simulink model "final_1EHA_comfiltro_V9"  (R2016a)
settings: Solver=FixedStepAuto  StartTime=72.65  StopTime=73.9  FixedStep=Ts  MaxStep=1e-7  RelTol=1e-4  AbsTol=1e-4
PreLoadFcn:
  | % -- Recommended Settings --
  | %
  | %  Simulink:
  | %      Solver: Ode23t
  | %      Relative tolerance = 1e-3
  | %       Max step size = 0.2
  | %
  | %  Powergui:
  |          Ts = 1e-07; % (discrete electrical model)
  | %
  | %  Control systems:
  |          Ts_control = 10*Ts; % (discrete control system)
  | %
  | % ----------------------------------
undefined symbols (not defined in the file or in its folder): C, L, R1, R2, sigbuilder_block
libraries: powerlib x92, dsparch4 x12, simulink x6, sps_avr x1, powerlib_meascontrol x1
(part 2 of 2)

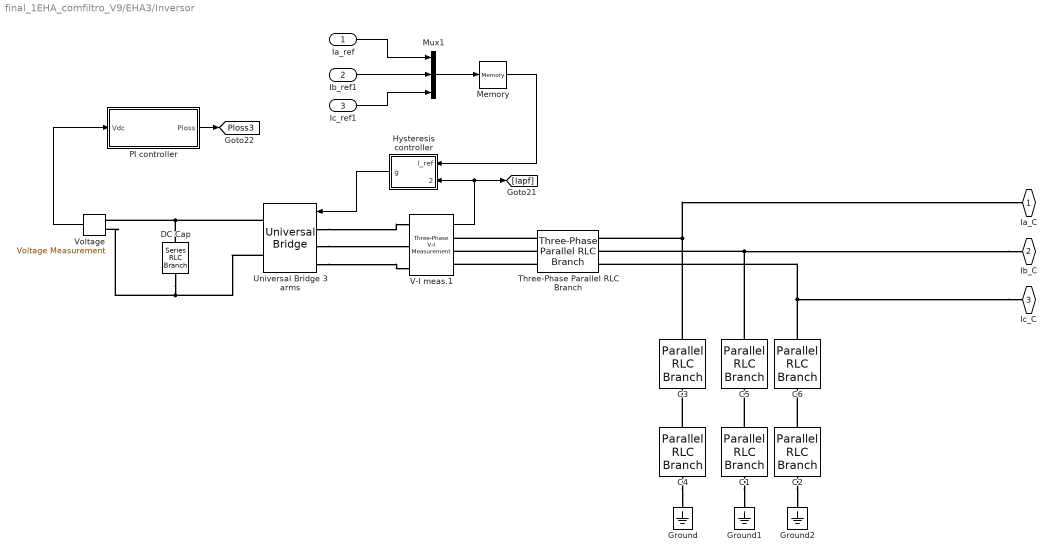
== system final_1EHA_comfiltro_V9/EHA3/Inversor ==
  Ia_ref : Inport
  Ib_ref1 : Inport  Port=2
  Ic_ref1 : Inport  Port=3
  C1 : powerlib/Elements/Parallel RLC Branch  LConnTagsString=a  RConnTagsString=__new0  BranchType=RC  Resistance=R2  Inductance=1e-3  SetiL0=off  InitialCurrent=0  Capacitance=C  Setx0=off  InitialVoltage=0  Measurements=None
  C2 : powerlib/Elements/Parallel RLC Branch  LConnTagsString=a  RConnTagsString=__new0  BranchType=RC  Resistance=R2  Inductance=1e-3  SetiL0=off  InitialCurrent=0  Capacitance=C  Setx0=off  InitialVoltage=0  Measurements=None
  C3 : powerlib/Elements/Parallel RLC Branch  LConnTagsString=a  RConnTagsString=__new0  BranchType=R  Resistance=R1  Inductance=1e-3  SetiL0=off  InitialCurrent=0  Capacitance=C  Setx0=off  InitialVoltage=0  Measurements=None
  C4 : powerlib/Elements/Parallel RLC Branch  LConnTagsString=a  RConnTagsString=__new0  BranchType=RC  Resistance=R2  Inductance=1e-3  SetiL0=off  InitialCurrent=0  Capacitance=C  Setx0=off  InitialVoltage=0  Measurements=None
  C5 : powerlib/Elements/Parallel RLC Branch  LConnTagsString=a  RConnTagsString=__new0  BranchType=R  Resistance=R1  Inductance=1e-3  SetiL0=off  InitialCurrent=0  Capacitance=C  Setx0=off  InitialVoltage=0  Measurements=None
  C6 : powerlib/Elements/Parallel RLC Branch  LConnTagsString=a  RConnTagsString=__new0  BranchType=R  Resistance=R1  Inductance=1e-3  SetiL0=off  InitialCurrent=0  Capacitance=C  Setx0=off  InitialVoltage=0  Measurements=None
  DC Cap : powerlib/Elements/Series RLC Branch  LConnTagsString=__new0  RConnTagsString=__new0  BranchType=C  Resistance=1  Inductance=1e-3  SetiL0=off  InitialCurrent=0  Capacitance=200e-6  Setx0=off  InitialVoltage=350  Measurements=None
  Ground : powerlib/Elements/Ground  LConnTagsString=a
  Ground1 : powerlib/Elements/Ground  LConnTagsString=a
  Ground2 : powerlib/Elements/Ground  LConnTagsString=a
  Hysteresis controller : Subsystem
  Memory : Memory
  Mux1 : Mux  Inputs=3
  PI controller : Subsystem
  Three-Phase Parallel RLC Branch : powerlib/Elements/Three-Phase Parallel RLC Branch  LConnTagsString=A|B|C  RConnTagsString=A|B|C  BranchType=L  Resistance=1  Inductance=L  Capacitance=1e-6  Measurements=None
  Universal Bridge 3 arms : powerlib/Power Electronics/Universal Bridge  Arms=3  SnubberResistance=1e8  SnubberCapacitance=inf  Device=Ideal Switches  Ron=1e-5  Lon=0  ForwardVoltages="[  1  1  ]"  ForwardVoltage=.8  GTOparameters=[ 10e-6 , 20e-6 ]  IGBTparameters=[ 1e-6 , 2e-6 ]  Measurements=None  Measurements_2=None  converterType=Rectifier
  V-I meas.1 : powerlib/Measurements/Three-Phase V-I Measurement  VoltageMeasurement=no  SetLabelV=off  LabelV=Vnm_EHA1  Vpu=off  VpuLL=off  CurrentMeasurement=yes  SetLabelI=off  LabelI=Iabc  Ipu=off  Pbase=100e6  Vbase=500e3  OutputType=Complex  PhasorSimulation=off  PSBequivalent=0
  Voltage : powerlib/Measurements/Voltage Measurement  PhasorSimulation=off  OutputType=Complex  PSBequivalent=0
  Ia_C : PMIOPort  Port=1  Side=Right
  Ib_C : PMIOPort  Port=2  Side=Right
  Ic_C : PMIOPort  Port=3  Side=Right
  tag scope: Ploss3=global
  wires:
  Voltage/1 -> PI controller/1(Vdc)
  PI controller/1(Ploss) -> [Ploss3]
  V-I meas.1/1 -> Hysteresis controller/2(I_meas), [Iapf]
  Mux1/1 -> Memory/1
  Hysteresis controller/1(g) -> Universal Bridge 3 arms/1
  Ia_ref/1 -> Mux1/1
  Ib_ref1/1 -> Mux1/2
  Ic_ref1/1 -> Mux1/3
  Memory/1 -> Hysteresis controller/1(I_ref)
  connections:
  Voltage/LConn1 -- Universal Bridge 3 arms/RConn1 -- DC Cap/LConn1
  Voltage/LConn2 -- Universal Bridge 3 arms/RConn2 -- DC Cap/RConn1
  Three-Phase Parallel RLC Branch/LConn2 -- V-I meas.1/RConn2
  Universal Bridge 3 arms/LConn1 -- V-I meas.1/LConn1
  Three-Phase Parallel RLC Branch/LConn1 -- V-I meas.1/RConn1
  Universal Bridge 3 arms/LConn2 -- V-I meas.1/LConn2
  Three-Phase Parallel RLC Branch/LConn3 -- V-I meas.1/RConn3
  Universal Bridge 3 arms/LConn3 -- V-I meas.1/LConn3
  Three-Phase Parallel RLC Branch/RConn1 -- C3/LConn1 -- Ia_C/RConn1
  Ib_C/RConn1 -- C5/LConn1 -- Three-Phase Parallel RLC Branch/RConn2
  Ic_C/RConn1 -- C6/LConn1 -- Three-Phase Parallel RLC Branch/RConn3
  C4/RConn1 -- Ground/LConn1
  C4/LConn1 -- C3/RConn1
  C2/LConn1 -- C6/RConn1
  C2/RConn1 -- Ground2/LConn1
  C1/LConn1 -- C5/RConn1
  C1/RConn1 -- Ground1/LConn1

== system final_1EHA_comfiltro_V9/EHA3/Signal Builder ==
  Demux : Demux  Tag=STV Demux  Outputs=1
  FromWs : FromWorkspace  Tag=STV FromWs  VariableName=tuvar  SampleTime=0
      SigBuilderData=|
      | common.afterFinalStr = 'Extrapolate'
      | common.sampleTime = 0
      | dataSet.timeRange = [72.75 73.9]
      | dataSet.name = 'Imported_Group 1'
      | sbobj.Name = 'Signal Builder'
      | sbobj.Groups.Name = 'Imported_Group 1'
      | sbobj.Groups.Signals.Name = 'var'
      | sbobj.Groups.Signals.XData = [72.75 72.751 72.752 72.753 72.754 72.755 72.756 72.757 72.758 72.759 72.76 72.761 ... (1151 elements, 1x1151)]
      | sbobj.Groups.Signals.YData = [0 0 0 0 0 0 0 0 0 0 0 0 ... (1151 elements, 1x1151)]
      | sbobj.Groups.TimeRange = [72.75 73.9]
  var : Outport
  wires:
  Demux/1 -> var/1
  FromWs/1 -> Demux/1

== system final_1EHA_comfiltro_V9/Primary Distribution (measurements & main contactor)/Contactor ==
  com : Inport
  Ideal Switch : powerlib/Power Electronics/Ideal Switch  Ron=0.001  Lon=0  IC=0  Rs=1e3  Cs=inf  Measurements=off
  Ideal Switch1 : powerlib/Power Electronics/Ideal Switch  Ron=0.001  Lon=0  IC=0  Rs=1e3  Cs=inf  Measurements=off
  Ideal Switch2 : powerlib/Power Electronics/Ideal Switch  Ron=0.001  Lon=0  IC=0  Rs=1e3  Cs=inf  Measurements=off
  A : PMIOPort  Port=1  Side=Left
  a : PMIOPort  Port=2  Side=Right
  B : PMIOPort  Port=3  Side=Left
  b : PMIOPort  Port=4  Side=Right
  C : PMIOPort  Port=5  Side=Left
  c : PMIOPort  Port=6  Side=Right
  wires:
  com/1 -> Ideal Switch1/1, Ideal Switch2/1, Ideal Switch/1
  connections:
  c/RConn1 -- Ideal Switch2/RConn1
  C/RConn1 -- Ideal Switch2/LConn1
  b/RConn1 -- Ideal Switch1/RConn1
  B/RConn1 -- Ideal Switch1/LConn1
  a/RConn1 -- Ideal Switch/RConn1
  A/RConn1 -- Ideal Switch/LConn1

== system final_1EHA_comfiltro_V9/EHA1/DSP/Calculo de potência Instantânea ==
  Ialpha' : Inport
  Ibeta' : Inport  Port=2
  valpha : Inport  Port=3
  vbeta : Inport  Port=4
  Fcn5 : Fcn  Expr=u(1)*u(3)+u(2)*u(4)
  Fcn6 : Fcn  Expr=u(2)*u(3)-u(1)*u(4)
  LPF : dsparch4/Analog Filter Design  method=Butterworth  filttype=Lowpass  N=5  Wlo=2*pi*200  Whi=80  Rp=2  Rs=40
  LPF1 : dsparch4/Analog Filter Design  method=Butterworth  filttype=Lowpass  N=5  Wlo=2*pi*200  Whi=80  Rp=2  Rs=40
  Mux2 : Mux
  pbarra' : Outport
  qbarra' : Outport  Port=2
  wires:
  Ibeta'/1 -> Mux2/4
  Ialpha'/1 -> Mux2/3
  LPF1/1 -> qbarra'/1
  LPF/1 -> pbarra'/1
  Mux2/1 -> Fcn6/1, Fcn5/1
  Fcn6/1 -> LPF1/1  "q'"
  Fcn5/1 -> LPF/1  "p'"
  vbeta/1 -> Mux2/2
  valpha/1 -> Mux2/1

== system final_1EHA_comfiltro_V9/EHA1/DSP/Cálculo de tensões alpha-beta ==
  Ialpha' : Inport
  Ibeta' : Inport  Port=2
  pbarra' : Inport  Port=3
  qbarra' : Inport  Port=4
  Add8 : Sum
  Divide5 : Product  Inputs=**
  Divide6 : Product  Inputs=**
  Divide8 : Product  Inputs=*/
  Divide9 : Product  Inputs=*/
  Fcn7 : Fcn  Expr=u(3)*u(1)-u(4)*u(2)
  Fcn8 : Fcn  Expr=u(4)*u(1)+u(3)*u(2)
  Gain8 : Gain
  Gain9 : Gain
  Mux6 : Mux
  valpha' : Outport
  vbeta' : Outport  Port=2
  wires:
  pbarra'/1 -> Gain8/1
  Divide5/1 -> Add8/1
  Divide6/1 -> Add8/2
  Gain8/1 -> Mux6/1
  Fcn8/1 -> Divide9/1
  Mux6/1 -> Fcn8/1, Fcn7/1
  qbarra'/1 -> Gain9/1
  Divide8/1 -> valpha'/1
  Fcn7/1 -> Divide8/1
  Gain9/1 -> Mux6/2
  Divide9/1 -> vbeta'/1
  Ibeta'/1 -> Mux6/4, Divide6/1, Divide6/2
  Ialpha'/1 -> Mux6/3, Divide5/1, Divide5/2
  Add8/1 -> Divide9/2, Divide8/2

== system final_1EHA_comfiltro_V9/EHA1/DSP/PLL ==
  Va : Inport
  Vb : Inport  Port=2
  Vc : Inport  Port=3
  Add10 : Sum
  Add3 : Sum  Inputs=+-
  Add4 : Sum  Inputs=+-
  Fcn1 : Fcn  Expr=sin(u(1))
  Fcn2 : Fcn  Expr=sin(u(1)+2*pi/3)
  Fcn3 : Fcn  Expr=sin(u(1)-pi/2)
  Fcn4 : Fcn  Expr=-cos(u(1)-pi/2)
  Integrator : Integrator
  PID Controller : simulink/Continuous/PID Controller  Controller=PI  TimeDomain=Continuous-time  SampleTime=-1  IntegratorMethod=Forward Euler  FilterMethod=Forward Euler  Form=Parallel  UseFilter=on  ControllerParametersSource=internal  P=25  I=22  D=0  N=100  InitialConditionSource=internal  InitialConditionForIntegrator=0  InitialConditionForFilter=0  ExternalReset=none  LimitOutput=off  UpperSaturationLimit=inf  LowerSaturationLimit=-inf  LinearizeAsGain=on  AntiWindupMode=none  Kb=1  TrackingMode=off  Kt=1  PParamMin=[]  PParamMax=[]  IParamMin=[]  IParamMax=[]  DParamMin=[]  DParamMax=[]  NParamMin=[]  NParamMax=[]  KbParamMin=[]  KbParamMax=[]  KtParamMin=[]  KtParamMax=[]  POutMin=[]  POutMax=[]  IOutMin=[]  IOutMax=[]  DOutMin=[]  DOutMax=[]  NOutMin=[]  NOutMax=[]  KbOutMin=[]  KbOutMax=[]  KtOutMin=[]  KtOutMax=[]  IntegratorOutMin=[]  IntegratorOutMax=[]  FilterOutMin=[]  FilterOutMax=[]  SumOutMin=[]  SumOutMax=[]  SumI1OutMin=[]  SumI1OutMax=[]  SumI2OutMin=[]  SumI2OutMax=[]  SumI3OutMin=[]  SumI3OutMax=[]  SumDOutMin=[]  SumDOutMax=[]  SaturationOutMin=[]  SaturationOutMax=[]  IntegratorContinuousStateAttributes=''  IntegratorStateMustResolveToSignalObject=off  IntegratorRTWStateStorageClass=Auto  FilterContinuousStateAttributes=''  FilterStateMustResolveToSignalObject=off  FilterRTWStateStorageClass=Auto  DifferentiatorICPrevScaledInput=0  DifferentiatorOutMin=[]  DifferentiatorOutMax=[]
  Product5 : Product
  Product6 : Product
  Ialpha' : Outport
  Ibeta' : Outport  Port=2
  wires:
  Va/1 -> Add3/1
  Add3/1 -> Product5/2  "Vab"
  Vc/1 -> Add4/1
  Fcn3/1 -> Ialpha'/1
  Fcn1/1 -> Product5/1
  Fcn2/1 -> Product6/2
  Integrator/1 -> Fcn2/1, Fcn4/1, Fcn1/1, Fcn3/1  "wt"
  Product6/1 -> Add10/2
  Vb/1 -> Add4/2, Add3/2
  Product5/1 -> Add10/1
  Add4/1 -> Product6/1  "Vcb"
  PID Controller/1 -> Integrator/1  "w"
  Add10/1 -> PID Controller/1  "P3phi"
  Fcn4/1 -> Ibeta'/1

== system final_1EHA_comfiltro_V9/EHA1/DSP/Subsystem ==
  Vabc' : Inport
  Iabc_L : Inport  Port=2
  Demux : Demux  Outputs=3
  Demux6 : Demux  Outputs=3
  Gain1 : Gain  Gain=sqrt(2/3)
  Gain2 : Gain  Gain=sqrt(2/3)
  Gain3 : Gain  Gain=[1/sqrt(2), 1/sqrt(2), 1/sqrt(2); 1, -1/2, -1/2; 0, sqrt(3)/2, -sqrt(3)/2]  Multiplication=Matrix(K*u)
  Gain4 : Gain  Gain=[1/sqrt(2), 1/sqrt(2), 1/sqrt(2); 1, -1/2, -1/2; 0, sqrt(3)/2, -sqrt(3)/2]  Multiplication=Matrix(K*u)
  Scope15 : Scope  NumInputPorts=2
  Terminator : Terminator
  Terminator1 : Terminator
  Valpha' : Outport
  Vbeta' : Outport  Port=2
  Ialpha : Outport  Port=3
  Ibeta : Outport  Port=4
  wires:
  Gain1/1 -> Gain3/1
  Gain2/1 -> Gain4/1
  Gain3/1 -> Demux/1, Scope15/1  "Valphabeta0"
  Demux/2 -> Valpha'/1  "Valpha"
  Demux6/2 -> Ialpha/1  "Ialpha"
  Demux/3 -> Vbeta'/1  "Vbeta"
  Demux6/3 -> Ibeta/1  "Ibeta"
  Iabc_L/1 -> Gain2/1
  Vabc'/1 -> Gain1/1
  Gain4/1 -> Demux6/1, Scope15/2  "Ialphabeta0"
  Demux6/1 -> Terminator/1  "I0"
  Demux/1 -> Terminator1/1  "V0"

== system final_1EHA_comfiltro_V9/EHA1/DSP/Subsystem1 ==
  Valpha' : Inport
  Vbeta' : Inport  Port=2
  Ialpha : Inport  Port=3
  Ibeta : Inport  Port=4
  Add : Sum
  Add10 : Sum
  Add3 : Sum  Inputs=+-
  Add4 : Sum  Inputs=+-
  LPF : dsparch4/Analog Filter Design  method=Butterworth  filttype=Lowpass  N=5  Wlo=2*pi*200  Whi=80  Rp=2  Rs=40
  Mux : Mux  Inputs=5
  Product{5..8} (4 alike) : Product
  Scope18 : Scope  NumInputPorts=5
  To Workspace : ToWorkspace  VariableName=p1  SaveFormat=Structure With Time  SampleTime=-1
  To Workspace1 : ToWorkspace  VariableName=q1  SaveFormat=Structure With Time  SampleTime=-1
  Posc : Outport
  q : Outport  Port=2
  wires:
  Product5/1 -> Add/1
  Product6/1 -> Add/2
  Add/1 -> Add4/2, LPF/1, Mux/1, Scope18/1  "P"
  Product7/1 -> Add3/1
  Product8/1 -> Add3/2
  Add3/1 -> To Workspace1/1, q/1  "q"
  LPF/1 -> Add4/1, Mux/2, Scope18/2  "Pbarra"
  Vbeta'/1 -> Product7/1, Product6/1
  Ialpha/1 -> Product7/2, Product5/2
  Valpha'/1 -> Product8/1, Product5/1
  Ibeta/1 -> Product8/2, Product6/2
  Add10/1 -> Posc/1, Scope18/5, Mux/5  "Posc"
  Add4/1 -> Scope18/3, Mux/3, Add10/2  "-Ptil"
  [Ploss1] -> Scope18/4, Mux/4, Add10/1  "Ploss"
  Mux/1 -> To Workspace/1

== system final_1EHA_comfiltro_V9/EHA1/DSP/Subsystem2 ==
  Valpha' : Inport
  Vbeta' : Inport  Port=2
  Posc : Inport  Port=3
  q : Inport  Port=4
  Add8 : Sum
  Add9 : Sum  Inputs=+-
  Divide{1..4} (4 alike) : Product  Inputs=***
  Fcn : Fcn  Expr=1/(u(1)^2+u(2)^2)
  Gain : Gain
  Gain5 : Gain  Gain=-1
  Mux : Mux  Inputs=2
  Scope20 : Scope  NumInputPorts=2
  Ialpha_p : Outport
  Ibeta_p : Outport  Port=2
  wires:
  Mux/1 -> Fcn/1
  Valpha'/1 -> Divide4/1, Mux/1, Divide1/1
  Vbeta'/1 -> Mux/2, Divide2/1, Divide3/1
  Posc/1 -> Gain5/1
  Fcn/1 -> Divide4/3, Divide3/3, Divide2/3, Divide1/3
  q/1 -> Gain/1
  Divide1/1 -> Add8/1
  Divide2/1 -> Add8/2
  Divide3/1 -> Add9/1
  Divide4/1 -> Add9/2
  Add9/1 -> Ibeta_p/1, Scope20/2  "Ibeta^*"
  Add8/1 -> Ialpha_p/1, Scope20/1  "Iaplha^*"
  Gain/1 -> Divide2/2, Divide4/2
  Gain5/1 -> Divide1/2, Divide3/2

== system final_1EHA_comfiltro_V9/EHA1/DSP/Subsystem3 ==
  Ialpha_p : Inport
  Ibeta_p : Inport  Port=2
  Fcn1 : Fcn  Expr=sqrt(2/3)*u(1)
  Fcn2 : Fcn  Expr=sqrt(2/3)*(-1/2*u(1)+sqrt(3)/2*u(2))
  Fcn3 : Fcn  Expr=sqrt(2/3)*(-1/2*u(1)-sqrt(3)/2*u(2))
  Mux2 : Mux  Inputs=2
  Mux3 : Mux  Inputs=2
  Mux5 : Mux  Inputs=2
  Scope14 : Scope  NumInputPorts=3
  Ia_C : Outport
  Ib_C : Outport  Port=2
  Ic_C : Outport  Port=3
  wires:
  Ibeta_p/1 -> Mux2/2, Mux3/2, Mux5/2
  Ialpha_p/1 -> Mux5/1, Mux2/1, Mux3/1
  Mux2/1 -> Fcn1/1
  Fcn1/1 -> Ia_C/1, Scope14/1  "Ia_C"
  Mux3/1 -> Fcn2/1
  Fcn2/1 -> Ib_C/1, Scope14/2  "Ib_C"
  Mux5/1 -> Fcn3/1
  Fcn3/1 -> Scope14/3, Ic_C/1  "Ic_C"

== system final_1EHA_comfiltro_V9/EHA1/DSP/TCT ==
  Va : Inport
  Vb : Inport  Port=2
  Vc : Inport  Port=3
  Demux7 : Demux  Outputs=3
  Gain1 : Gain  Gain=sqrt(2/3)
  Gain3 : Gain  Gain=[1/sqrt(2), 1/sqrt(2), 1/sqrt(2); 1, -1/2, -1/2; 0, sqrt(3)/2, -sqrt(3)/2]  Multiplication=Matrix(K*u)
  Mux2 : Mux  Inputs=3
  valpha : Outport
  vbeta : Outport  Port=2
  wires:
  Gain3/1 -> Demux7/1  "Valphabeta0"
  Gain1/1 -> Gain3/1
  Mux2/1 -> Gain1/1
  Va/1 -> Mux2/1
  Vb/1 -> Mux2/2
  Vc/1 -> Mux2/3
  Demux7/2 -> valpha/1
  Demux7/3 -> vbeta/1

== system final_1EHA_comfiltro_V9/EHA1/DSP/Transformada Inversa de Clarke ==
  valpha' : Inport
  vbeta' : Inport  Port=2
  Demux6 : Demux  Outputs=3
  Fcn10 : Fcn  Expr=sqrt(2/3)*(-1/2*u(1)+sqrt(3)/2*u(2))
  Fcn11 : Fcn  Expr=sqrt(2/3)*(-1/2*u(1)-sqrt(3)/2*u(2))
  Fcn9 : Fcn  Expr=sqrt(2/3)*(u(1) + 0*u(2))
  Mux{3,5,8..9} (4 alike) : Mux  Inputs=2
  Scope23 : Scope  NumInputPorts=3
  va' : Outport
  vb' : Outport  Port=2
  vc' : Outport  Port=3
  wires:
  Fcn10/1 -> vb'/1, Scope23/2  "vb'"
  Demux6/1 -> Mux9/1
  valpha'/1 -> Mux5/1, Mux8/1, Mux3/1
  vbeta'/1 -> Mux3/2, Mux5/2, Mux8/2
  Mux5/1 -> Fcn10/1
  Mux3/1 -> Fcn9/1
  Fcn11/1 -> vc'/1, Scope23/3  "vc'"
  Fcn9/1 -> va'/1, Mux9/2  "va'"
  Mux8/1 -> Fcn11/1
  [Vabc_S] -> Demux6/1
  Mux9/1 -> Scope23/1

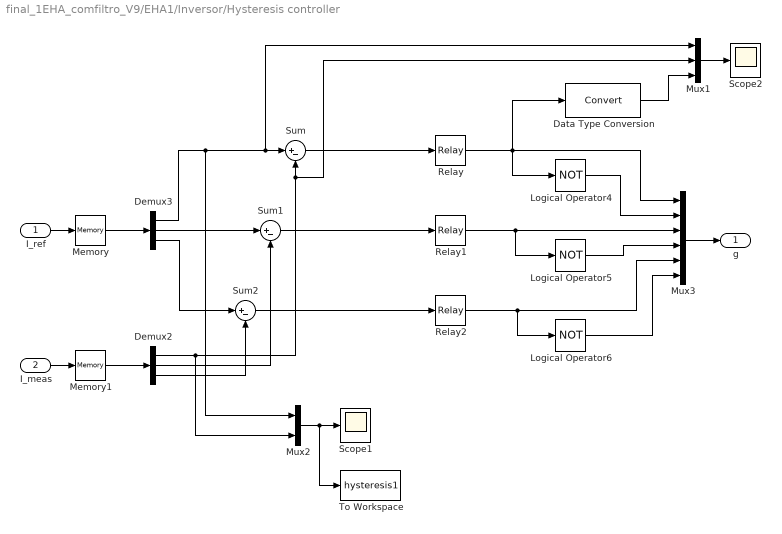
== system final_1EHA_comfiltro_V9/EHA1/Inversor/Hysteresis controller ==
  I_ref : Inport
  I_meas : Inport  Port=2
  Data Type Conversion : DataTypeConversion
  Demux2 : Demux  Outputs=3
  Demux3 : Demux  Outputs=3
  Logical Operator4 : Logic  Operator=NOT  AllPortsSameDT=off  OutDataTypeStr=boolean
  Logical Operator5 : Logic  Operator=NOT  AllPortsSameDT=off  OutDataTypeStr=boolean
  Logical Operator6 : Logic  Operator=NOT  AllPortsSameDT=off  OutDataTypeStr=boolean
  Memory : Memory
  Memory1 : Memory
  Mux1 : Mux  Inputs=3
  Mux2 : Mux  Inputs=2
  Mux3 : Mux  Inputs=6
  Relay : Relay  OnSwitchValue=0.05  OffSwitchValue=-0.05  OutDataTypeStr=Inherit: Inherit via back propagation
  Relay1 : Relay  OnSwitchValue=0.05  OffSwitchValue=-0.05  OutDataTypeStr=Inherit: Inherit via back propagation
  Relay2 : Relay  OnSwitchValue=0.05  OffSwitchValue=-0.05  OutDataTypeStr=Inherit: Inherit via back propagation
  Scope1 : Scope
  Scope2 : Scope
  Sum : Sum  Inputs=|+-
  Sum1 : Sum  Inputs=|+-
  Sum2 : Sum  Inputs=|+-
  To Workspace : ToWorkspace  VariableName=hysteresis1  SaveFormat=Structure With Time  SampleTime=-1
  g : Outport
  wires:
  I_ref/1 -> Memory/1
  I_meas/1 -> Memory1/1
  Relay1/1 -> Logical Operator5/1, Mux3/3
  Demux3/1 -> Mux1/1, Sum/1, Mux2/1
  Logical Operator4/1 -> Mux3/2
  Logical Operator5/1 -> Mux3/4
  Logical Operator6/1 -> Mux3/6
  Mux3/1 -> g/1
  Demux2/1 -> Mux2/2, Mux1/2, Sum/2
  Memory/1 -> Demux3/1
  Memory1/1 -> Demux2/1
  Mux2/1 -> To Workspace/1, Scope1/1
  Relay/1 -> Data Type Conversion/1, Mux3/1, Logical Operator4/1
  Demux3/2 -> Sum1/1
  Demux2/2 -> Sum1/2
  Demux3/3 -> Sum2/1
  Demux2/3 -> Sum2/2
  Relay2/1 -> Mux3/5, Logical Operator6/1
  Mux1/1 -> Scope2/1
  Data Type Conversion/1 -> Mux1/3
  Sum/1 -> Relay/1
  Sum1/1 -> Relay1/1
  Sum2/1 -> Relay2/1

== system final_1EHA_comfiltro_V9/EHA1/Inversor/PI controller ==
  Vdc : Inport
  LPF : dsparch4/Analog Filter Design  method=Butterworth  filttype=Lowpass  N=5  Wlo=2*pi*200  Whi=80  Rp=2  Rs=40
  PID Controller : simulink/Continuous/PID Controller  Controller=PI  TimeDomain=Continuous-time  SampleTime=-1  IntegratorMethod=Forward Euler  FilterMethod=Forward Euler  Form=Ideal  UseFilter=on  ControllerParametersSource=internal  P=5  I=7  D=0  N=100  InitialConditionSource=internal  InitialConditionForIntegrator=0  InitialConditionForFilter=0  ExternalReset=none  LimitOutput=off  UpperSaturationLimit=inf  LowerSaturationLimit=-inf  LinearizeAsGain=on  AntiWindupMode=none  Kb=1  TrackingMode=off  Kt=1  PParamMin=[]  PParamMax=[]  IParamMin=[]  IParamMax=[]  DParamMin=[]  DParamMax=[]  NParamMin=[]  NParamMax=[]  KbParamMin=[]  KbParamMax=[]  KtParamMin=[]  KtParamMax=[]  POutMin=[]  POutMax=[]  IOutMin=[]  IOutMax=[]  DOutMin=[]  DOutMax=[]  NOutMin=[]  NOutMax=[]  KbOutMin=[]  KbOutMax=[]  KtOutMin=[]  KtOutMax=[]  IntegratorOutMin=[]  IntegratorOutMax=[]  FilterOutMin=[]  FilterOutMax=[]  SumOutMin=[]  SumOutMax=[]  SumI1OutMin=[]  SumI1OutMax=[]  SumI2OutMin=[]  SumI2OutMax=[]  SumI3OutMin=[]  SumI3OutMax=[]  SumDOutMin=[]  SumDOutMax=[]  SaturationOutMin=[]  SaturationOutMax=[]  IntegratorContinuousStateAttributes=''  IntegratorStateMustResolveToSignalObject=off  IntegratorRTWStateStorageClass=Auto  FilterContinuousStateAttributes=''  FilterStateMustResolveToSignalObject=off  FilterRTWStateStorageClass=Auto  DifferentiatorICPrevScaledInput=0  DifferentiatorOutMin=[]  DifferentiatorOutMax=[]
  Scope : Scope  NumInputPorts=3
  Signal Builder1 : Subsystem  Tag=STV Subsys  LoadFcn=sigbuilder_block('load');  StartFcn=sigbuilder_block('start');  StopFcn=sigbuilder_block('stop');  ClipboardFcn=sigbuilder_block('clipboard');  mask(Sigbuilder block){}
      mask help: Simulink:masks:SigbuilderBlock_MD
      mask init:
      | if ~strcmp(get_param(bdroot(gcbh),'SimulationStatus'),'stopped') tuvar = sigbuilder_block('maskInit'); end
      settings: CopyFcn=sigbuilder_block('copy');  DeleteFcn=sigbuilder_block('delete');  ModelCloseFcn=sigbuilder_block('modelClose');  PreSaveFcn=sigbuilder_block('preSave');  PauseFcn=sigbuilder_block('pause');  ContinueFcn=sigbuilder_block('continue');  NameChangeFcn=sigbuilder_block('namechange');  OpenFcn=sigbuilder_block('open',[437.6 199.2 550.4 400 ]);  CloseFcn=sigbuilder_block('close');
      mask Display: plot(0, 0, 100, 100,[2, 2, 32, 32, 2], [68, 8, 8, 68, 68],[32, 2], [38, 38], [32, 19, 2],[53, 60, 44], [32, 17, 17, 2],[16, 16, 31, 31]);txt = getActiveGroup(gcbh);text(2, 100, txt,'verticalAlignment', 'top');
  Sum : Sum  Inputs=|-+
  Ploss : Outport
  wires:
  Vdc/1 -> Scope/1, Sum/1  "Vdc1"
  Sum/1 -> Scope/2, LPF/1  "Vdc1-step"
  Signal Builder1/1(Signal 1) -> Sum/2
  LPF/1 -> PID Controller/1
  PID Controller/1 -> Scope/3, Ploss/1

== system final_1EHA_comfiltro_V9/EHA2/DSP/Calculo de potência Instantânea ==
  Ialpha' : Inport
  Ibeta' : Inport  Port=2
  valpha : Inport  Port=3
  vbeta : Inport  Port=4
  Fcn5 : Fcn  Expr=u(1)*u(3)+u(2)*u(4)
  Fcn6 : Fcn  Expr=u(2)*u(3)-u(1)*u(4)
  LPF : dsparch4/Analog Filter Design  method=Butterworth  filttype=Lowpass  N=5  Wlo=2*pi*200  Whi=80  Rp=2  Rs=40
  LPF1 : dsparch4/Analog Filter Design  method=Butterworth  filttype=Lowpass  N=5  Wlo=2*pi*200  Whi=80  Rp=2  Rs=40
  Mux2 : Mux
  pbarra' : Outport
  qbarra' : Outport  Port=2
  wires:
  Ibeta'/1 -> Mux2/4
  Ialpha'/1 -> Mux2/3
  LPF1/1 -> qbarra'/1
  LPF/1 -> pbarra'/1
  Mux2/1 -> Fcn6/1, Fcn5/1
  Fcn6/1 -> LPF1/1  "q'"
  Fcn5/1 -> LPF/1  "p'"
  vbeta/1 -> Mux2/2
  valpha/1 -> Mux2/1

== system final_1EHA_comfiltro_V9/EHA2/DSP/Cálculo de tensões alpha-beta ==
  Ialpha' : Inport
  Ibeta' : Inport  Port=2
  pbarra' : Inport  Port=3
  qbarra' : Inport  Port=4
  Add8 : Sum
  Divide5 : Product  Inputs=**
  Divide6 : Product  Inputs=**
  Divide8 : Product  Inputs=*/
  Divide9 : Product  Inputs=*/
  Fcn7 : Fcn  Expr=u(3)*u(1)-u(4)*u(2)
  Fcn8 : Fcn  Expr=u(4)*u(1)+u(3)*u(2)
  Gain8 : Gain
  Gain9 : Gain
  Mux6 : Mux
  valpha' : Outport
  vbeta' : Outport  Port=2
  wires:
  pbarra'/1 -> Gain8/1
  Divide5/1 -> Add8/1
  Divide6/1 -> Add8/2
  Gain8/1 -> Mux6/1
  Fcn8/1 -> Divide9/1
  Mux6/1 -> Fcn8/1, Fcn7/1
  qbarra'/1 -> Gain9/1
  Divide8/1 -> valpha'/1
  Fcn7/1 -> Divide8/1
  Gain9/1 -> Mux6/2
  Divide9/1 -> vbeta'/1
  Ibeta'/1 -> Mux6/4, Divide6/1, Divide6/2
  Ialpha'/1 -> Mux6/3, Divide5/1, Divide5/2
  Add8/1 -> Divide9/2, Divide8/2

== system final_1EHA_comfiltro_V9/EHA2/DSP/PLL ==
  Va : Inport
  Vb : Inport  Port=2
  Vc : Inport  Port=3
  Add10 : Sum
  Add3 : Sum  Inputs=+-
  Add4 : Sum  Inputs=+-
  Fcn1 : Fcn  Expr=sin(u(1))
  Fcn2 : Fcn  Expr=sin(u(1)+2*pi/3)
  Fcn3 : Fcn  Expr=sin(u(1)-pi/2)
  Fcn4 : Fcn  Expr=-cos(u(1)-pi/2)
  Integrator : Integrator
  PID Controller : simulink/Continuous/PID Controller  Controller=PI  TimeDomain=Continuous-time  SampleTime=-1  IntegratorMethod=Forward Euler  FilterMethod=Forward Euler  Form=Parallel  UseFilter=on  ControllerParametersSource=internal  P=25  I=22  D=0  N=100  InitialConditionSource=internal  InitialConditionForIntegrator=0  InitialConditionForFilter=0  ExternalReset=none  LimitOutput=off  UpperSaturationLimit=inf  LowerSaturationLimit=-inf  LinearizeAsGain=on  AntiWindupMode=none  Kb=1  TrackingMode=off  Kt=1  PParamMin=[]  PParamMax=[]  IParamMin=[]  IParamMax=[]  DParamMin=[]  DParamMax=[]  NParamMin=[]  NParamMax=[]  KbParamMin=[]  KbParamMax=[]  KtParamMin=[]  KtParamMax=[]  POutMin=[]  POutMax=[]  IOutMin=[]  IOutMax=[]  DOutMin=[]  DOutMax=[]  NOutMin=[]  NOutMax=[]  KbOutMin=[]  KbOutMax=[]  KtOutMin=[]  KtOutMax=[]  IntegratorOutMin=[]  IntegratorOutMax=[]  FilterOutMin=[]  FilterOutMax=[]  SumOutMin=[]  SumOutMax=[]  SumI1OutMin=[]  SumI1OutMax=[]  SumI2OutMin=[]  SumI2OutMax=[]  SumI3OutMin=[]  SumI3OutMax=[]  SumDOutMin=[]  SumDOutMax=[]  SaturationOutMin=[]  SaturationOutMax=[]  IntegratorContinuousStateAttributes=''  IntegratorStateMustResolveToSignalObject=off  IntegratorRTWStateStorageClass=Auto  FilterContinuousStateAttributes=''  FilterStateMustResolveToSignalObject=off  FilterRTWStateStorageClass=Auto  DifferentiatorICPrevScaledInput=0  DifferentiatorOutMin=[]  DifferentiatorOutMax=[]
  Product5 : Product
  Product6 : Product
  Ialpha' : Outport
  Ibeta' : Outport  Port=2
  wires:
  Va/1 -> Add3/1
  Add3/1 -> Product5/2  "Vab"
  Vc/1 -> Add4/1
  Fcn3/1 -> Ialpha'/1
  Fcn1/1 -> Product5/1
  Fcn2/1 -> Product6/2
  Integrator/1 -> Fcn2/1, Fcn4/1, Fcn1/1, Fcn3/1  "wt"
  Product6/1 -> Add10/2
  Vb/1 -> Add4/2, Add3/2
  Product5/1 -> Add10/1
  Add4/1 -> Product6/1  "Vcb"
  PID Controller/1 -> Integrator/1  "w"
  Add10/1 -> PID Controller/1  "P3phi"
  Fcn4/1 -> Ibeta'/1

== system final_1EHA_comfiltro_V9/EHA2/DSP/Subsystem ==
  Vabc' : Inport
  Iabc_L : Inport  Port=2
  Demux : Demux  Outputs=3
  Demux6 : Demux  Outputs=3
  Gain1 : Gain  Gain=sqrt(2/3)
  Gain2 : Gain  Gain=sqrt(2/3)
  Gain3 : Gain  Gain=[1/sqrt(2), 1/sqrt(2), 1/sqrt(2); 1, -1/2, -1/2; 0, sqrt(3)/2, -sqrt(3)/2]  Multiplication=Matrix(K*u)
  Gain4 : Gain  Gain=[1/sqrt(2), 1/sqrt(2), 1/sqrt(2); 1, -1/2, -1/2; 0, sqrt(3)/2, -sqrt(3)/2]  Multiplication=Matrix(K*u)
  Scope15 : Scope  NumInputPorts=2
  Terminator : Terminator
  Terminator1 : Terminator
  Valpha' : Outport
  Vbeta' : Outport  Port=2
  Ialpha : Outport  Port=3
  Ibeta : Outport  Port=4
  wires:
  Gain1/1 -> Gain3/1
  Gain2/1 -> Gain4/1
  Gain3/1 -> Demux/1, Scope15/1  "Valphabeta0"
  Demux/2 -> Valpha'/1  "Valpha"
  Demux6/2 -> Ialpha/1  "Ialpha"
  Demux/3 -> Vbeta'/1  "Vbeta"
  Demux6/3 -> Ibeta/1  "Ibeta"
  Iabc_L/1 -> Gain2/1
  Vabc'/1 -> Gain1/1
  Gain4/1 -> Demux6/1, Scope15/2  "Ialphabeta0"
  Demux6/1 -> Terminator/1  "I0"
  Demux/1 -> Terminator1/1  "V0"

== system final_1EHA_comfiltro_V9/EHA2/DSP/Subsystem1 ==
  Valpha' : Inport
  Vbeta' : Inport  Port=2
  Ialpha : Inport  Port=3
  Ibeta : Inport  Port=4
  Add : Sum
  Add10 : Sum
  Add3 : Sum  Inputs=+-
  Add4 : Sum  Inputs=+-
  LPF : dsparch4/Analog Filter Design  method=Butterworth  filttype=Lowpass  N=5  Wlo=2*pi*200  Whi=80  Rp=2  Rs=40
  Product{5..8} (4 alike) : Product
  Scope18 : Scope  NumInputPorts=5
  Posc : Outport
  q : Outport  Port=2
  wires:
  Product5/1 -> Add/1
  Product6/1 -> Add/2
  Add/1 -> Add4/2, LPF/1, Scope18/1  "P"
  Product7/1 -> Add3/1
  Product8/1 -> Add3/2
  Add3/1 -> q/1  "q"
  LPF/1 -> Add4/1, Scope18/2  "Pbarra"
  Vbeta'/1 -> Product7/1, Product6/1
  Ialpha/1 -> Product7/2, Product5/2
  Valpha'/1 -> Product8/1, Product5/1
  Ibeta/1 -> Product8/2, Product6/2
  Add10/1 -> Posc/1, Scope18/5  "Posc"
  Add4/1 -> Scope18/3, Add10/2  "-Ptil"
  [Ploss2] -> Scope18/4, Add10/1  "Ploss"

== system final_1EHA_comfiltro_V9/EHA2/DSP/Subsystem2 ==
  Valpha' : Inport
  Vbeta' : Inport  Port=2
  Posc : Inport  Port=3
  q : Inport  Port=4
  Add8 : Sum
  Add9 : Sum  Inputs=+-
  Divide{1..4} (4 alike) : Product  Inputs=***
  Fcn : Fcn  Expr=1/(u(1)^2+u(2)^2)
  Gain : Gain
  Gain5 : Gain  Gain=-1
  Mux : Mux  Inputs=2
  Scope20 : Scope  NumInputPorts=2
  Ialpha_p : Outport
  Ibeta_p : Outport  Port=2
  wires:
  Mux/1 -> Fcn/1
  Valpha'/1 -> Divide4/1, Mux/1, Divide1/1
  Vbeta'/1 -> Mux/2, Divide2/1, Divide3/1
  Posc/1 -> Gain5/1
  Fcn/1 -> Divide4/3, Divide3/3, Divide2/3, Divide1/3
  q/1 -> Gain/1
  Divide1/1 -> Add8/1
  Divide2/1 -> Add8/2
  Divide3/1 -> Add9/1
  Divide4/1 -> Add9/2
  Add9/1 -> Ibeta_p/1, Scope20/2  "Ibeta^*"
  Add8/1 -> Ialpha_p/1, Scope20/1  "Iaplha^*"
  Gain/1 -> Divide2/2, Divide4/2
  Gain5/1 -> Divide1/2, Divide3/2

== system final_1EHA_comfiltro_V9/EHA2/DSP/Subsystem3 ==
  Ialpha_p : Inport
  Ibeta_p : Inport  Port=2
  Fcn1 : Fcn  Expr=sqrt(2/3)*u(1)
  Fcn2 : Fcn  Expr=sqrt(2/3)*(-1/2*u(1)+sqrt(3)/2*u(2))
  Fcn3 : Fcn  Expr=sqrt(2/3)*(-1/2*u(1)-sqrt(3)/2*u(2))
  Mux2 : Mux  Inputs=2
  Mux3 : Mux  Inputs=2
  Mux5 : Mux  Inputs=2
  Scope14 : Scope  NumInputPorts=3
  Ia_C : Outport
  Ib_C : Outport  Port=2
  Ic_C : Outport  Port=3
  wires:
  Ibeta_p/1 -> Mux2/2, Mux3/2, Mux5/2
  Ialpha_p/1 -> Mux5/1, Mux2/1, Mux3/1
  Mux2/1 -> Fcn1/1
  Fcn1/1 -> Ia_C/1, Scope14/1  "Ia_C"
  Mux3/1 -> Fcn2/1
  Fcn2/1 -> Ib_C/1, Scope14/2  "Ib_C"
  Mux5/1 -> Fcn3/1
  Fcn3/1 -> Scope14/3, Ic_C/1  "Ic_C"

== system final_1EHA_comfiltro_V9/EHA2/DSP/TCT ==
  Va : Inport
  Vb : Inport  Port=2
  Vc : Inport  Port=3
  Demux7 : Demux  Outputs=3
  Gain1 : Gain  Gain=sqrt(2/3)
  Gain3 : Gain  Gain=[1/sqrt(2), 1/sqrt(2), 1/sqrt(2); 1, -1/2, -1/2; 0, sqrt(3)/2, -sqrt(3)/2]  Multiplication=Matrix(K*u)
  Mux2 : Mux  Inputs=3
  valpha : Outport
  vbeta : Outport  Port=2
  wires:
  Gain3/1 -> Demux7/1  "Valphabeta0"
  Gain1/1 -> Gain3/1
  Mux2/1 -> Gain1/1
  Va/1 -> Mux2/1
  Vb/1 -> Mux2/2
  Vc/1 -> Mux2/3
  Demux7/2 -> valpha/1
  Demux7/3 -> vbeta/1

== system final_1EHA_comfiltro_V9/EHA2/DSP/Transformada Inversa de Clarke ==
  valpha' : Inport
  vbeta' : Inport  Port=2
  Demux6 : Demux  Outputs=3
  Fcn10 : Fcn  Expr=sqrt(2/3)*(-1/2*u(1)+sqrt(3)/2*u(2))
  Fcn11 : Fcn  Expr=sqrt(2/3)*(-1/2*u(1)-sqrt(3)/2*u(2))
  Fcn9 : Fcn  Expr=sqrt(2/3)*(u(1) + 0*u(2))
  Mux{3,5,8..9} (4 alike) : Mux  Inputs=2
  Scope23 : Scope  NumInputPorts=3
  va' : Outport
  vb' : Outport  Port=2
  vc' : Outport  Port=3
  wires:
  Fcn10/1 -> vb'/1, Scope23/2  "vb'"
  Demux6/1 -> Mux9/1
  valpha'/1 -> Mux5/1, Mux8/1, Mux3/1
  vbeta'/1 -> Mux3/2, Mux5/2, Mux8/2
  Mux5/1 -> Fcn10/1
  Mux3/1 -> Fcn9/1
  Fcn11/1 -> vc'/1, Scope23/3  "vc'"
  Fcn9/1 -> va'/1, Mux9/2  "va'"
  Mux8/1 -> Fcn11/1
  [Vabc_S] -> Demux6/1
  Mux9/1 -> Scope23/1

== system final_1EHA_comfiltro_V9/EHA2/Inversor/Hysteresis controller ==
  I_ref : Inport
  I_meas : Inport  Port=2
  Demux2 : Demux  Outputs=3
  Demux3 : Demux  Outputs=3
  Logical Operator4 : Logic  Operator=NOT  AllPortsSameDT=off  OutDataTypeStr=boolean
  Logical Operator5 : Logic  Operator=NOT  AllPortsSameDT=off  OutDataTypeStr=boolean
  Logical Operator6 : Logic  Operator=NOT  AllPortsSameDT=off  OutDataTypeStr=boolean
  Memory : Memory
  Memory1 : Memory
  Mux3 : Mux  Inputs=6
  Relay : Relay  OnSwitchValue=0.05  OffSwitchValue=-0.05  OutDataTypeStr=Inherit: Inherit via back propagation
  Relay1 : Relay  OnSwitchValue=0.05  OffSwitchValue=-0.05  OutDataTypeStr=Inherit: Inherit via back propagation
  Relay2 : Relay  OnSwitchValue=0.05  OffSwitchValue=-0.05  OutDataTypeStr=Inherit: Inherit via back propagation
  Sum : Sum  Inputs=|+-
  Sum1 : Sum  Inputs=|+-
  Sum2 : Sum  Inputs=|+-
  g : Outport
  wires:
  I_ref/1 -> Memory/1
  I_meas/1 -> Memory1/1
  Relay1/1 -> Logical Operator5/1, Mux3/3
  Demux3/1 -> Sum/1
  Logical Operator4/1 -> Mux3/2
  Logical Operator5/1 -> Mux3/4
  Logical Operator6/1 -> Mux3/6
  Mux3/1 -> g/1
  Demux2/1 -> Sum/2
  Memory/1 -> Demux3/1
  Memory1/1 -> Demux2/1
  Relay/1 -> Mux3/1, Logical Operator4/1
  Demux3/2 -> Sum1/1
  Demux2/2 -> Sum1/2
  Demux3/3 -> Sum2/1
  Demux2/3 -> Sum2/2
  Relay2/1 -> Mux3/5, Logical Operator6/1
  Sum/1 -> Relay/1
  Sum1/1 -> Relay1/1
  Sum2/1 -> Relay2/1

== system final_1EHA_comfiltro_V9/EHA2/Inversor/PI controller ==
  Vdc : Inport
  LPF : dsparch4/Analog Filter Design  method=Butterworth  filttype=Lowpass  N=5  Wlo=2*pi*200  Whi=80  Rp=2  Rs=40
  PID Controller : simulink/Continuous/PID Controller  Controller=PI  TimeDomain=Continuous-time  SampleTime=-1  IntegratorMethod=Forward Euler  FilterMethod=Forward Euler  Form=Ideal  UseFilter=on  ControllerParametersSource=internal  P=5  I=7  D=0  N=100  InitialConditionSource=internal  InitialConditionForIntegrator=0  InitialConditionForFilter=0  ExternalReset=none  LimitOutput=off  UpperSaturationLimit=inf  LowerSaturationLimit=-inf  LinearizeAsGain=on  AntiWindupMode=none  Kb=1  TrackingMode=off  Kt=1  PParamMin=[]  PParamMax=[]  IParamMin=[]  IParamMax=[]  DParamMin=[]  DParamMax=[]  NParamMin=[]  NParamMax=[]  KbParamMin=[]  KbParamMax=[]  KtParamMin=[]  KtParamMax=[]  POutMin=[]  POutMax=[]  IOutMin=[]  IOutMax=[]  DOutMin=[]  DOutMax=[]  NOutMin=[]  NOutMax=[]  KbOutMin=[]  KbOutMax=[]  KtOutMin=[]  KtOutMax=[]  IntegratorOutMin=[]  IntegratorOutMax=[]  FilterOutMin=[]  FilterOutMax=[]  SumOutMin=[]  SumOutMax=[]  SumI1OutMin=[]  SumI1OutMax=[]  SumI2OutMin=[]  SumI2OutMax=[]  SumI3OutMin=[]  SumI3OutMax=[]  SumDOutMin=[]  SumDOutMax=[]  SaturationOutMin=[]  SaturationOutMax=[]  IntegratorContinuousStateAttributes=''  IntegratorStateMustResolveToSignalObject=off  IntegratorRTWStateStorageClass=Auto  FilterContinuousStateAttributes=''  FilterStateMustResolveToSignalObject=off  FilterRTWStateStorageClass=Auto  DifferentiatorICPrevScaledInput=0  DifferentiatorOutMin=[]  DifferentiatorOutMax=[]
  Scope : Scope  NumInputPorts=3
  Signal Builder1 : Subsystem  Tag=STV Subsys  LoadFcn=sigbuilder_block('load');  StartFcn=sigbuilder_block('start');  StopFcn=sigbuilder_block('stop');  ClipboardFcn=sigbuilder_block('clipboard');  mask(Sigbuilder block){}
      mask help: Simulink:masks:SigbuilderBlock_MD
      mask init:
      | if ~strcmp(get_param(bdroot(gcbh),'SimulationStatus'),'stopped') tuvar = sigbuilder_block('maskInit'); end
      settings: CopyFcn=sigbuilder_block('copy');  DeleteFcn=sigbuilder_block('delete');  ModelCloseFcn=sigbuilder_block('modelClose');  PreSaveFcn=sigbuilder_block('preSave');  PauseFcn=sigbuilder_block('pause');  ContinueFcn=sigbuilder_block('continue');  NameChangeFcn=sigbuilder_block('namechange');  OpenFcn=sigbuilder_block('open',[437.6 199.2 550.4 400 ]);  CloseFcn=sigbuilder_block('close');
      mask Display: plot(0, 0, 100, 100,[2, 2, 32, 32, 2], [68, 8, 8, 68, 68],[32, 2], [38, 38], [32, 19, 2],[53, 60, 44], [32, 17, 17, 2],[16, 16, 31, 31]);txt = getActiveGroup(gcbh);text(2, 100, txt,'verticalAlignment', 'top');
  Sum : Sum  Inputs=|-+
  Ploss : Outport
  wires:
  Vdc/1 -> Scope/1, Sum/1  "Vdc1"
  Sum/1 -> Scope/2, LPF/1  "Vdc1-step"
  Signal Builder1/1(Signal 1) -> Sum/2
  LPF/1 -> PID Controller/1
  PID Controller/1 -> Scope/3, Ploss/1

== system final_1EHA_comfiltro_V9/EHA3/DSP/Calculo de potência Instantânea ==
  Ialpha' : Inport
  Ibeta' : Inport  Port=2
  valpha : Inport  Port=3
  vbeta : Inport  Port=4
  Fcn5 : Fcn  Expr=u(1)*u(3)+u(2)*u(4)
  Fcn6 : Fcn  Expr=u(2)*u(3)-u(1)*u(4)
  LPF : dsparch4/Analog Filter Design  method=Butterworth  filttype=Lowpass  N=5  Wlo=2*pi*200  Whi=80  Rp=2  Rs=40
  LPF1 : dsparch4/Analog Filter Design  method=Butterworth  filttype=Lowpass  N=5  Wlo=2*pi*200  Whi=80  Rp=2  Rs=40
  Mux2 : Mux
  pbarra' : Outport
  qbarra' : Outport  Port=2
  wires:
  Ibeta'/1 -> Mux2/4
  Ialpha'/1 -> Mux2/3
  LPF1/1 -> qbarra'/1
  LPF/1 -> pbarra'/1
  Mux2/1 -> Fcn6/1, Fcn5/1
  Fcn6/1 -> LPF1/1  "q'"
  Fcn5/1 -> LPF/1  "p'"
  vbeta/1 -> Mux2/2
  valpha/1 -> Mux2/1

== system final_1EHA_comfiltro_V9/EHA3/DSP/Cálculo de tensões alpha-beta ==
  Ialpha' : Inport
  Ibeta' : Inport  Port=2
  pbarra' : Inport  Port=3
  qbarra' : Inport  Port=4
  Add8 : Sum
  Divide5 : Product  Inputs=**
  Divide6 : Product  Inputs=**
  Divide8 : Product  Inputs=*/
  Divide9 : Product  Inputs=*/
  Fcn7 : Fcn  Expr=u(3)*u(1)-u(4)*u(2)
  Fcn8 : Fcn  Expr=u(4)*u(1)+u(3)*u(2)
  Gain8 : Gain
  Gain9 : Gain
  Mux6 : Mux
  valpha' : Outport
  vbeta' : Outport  Port=2
  wires:
  pbarra'/1 -> Gain8/1
  Divide5/1 -> Add8/1
  Divide6/1 -> Add8/2
  Gain8/1 -> Mux6/1
  Fcn8/1 -> Divide9/1
  Mux6/1 -> Fcn8/1, Fcn7/1
  qbarra'/1 -> Gain9/1
  Divide8/1 -> valpha'/1
  Fcn7/1 -> Divide8/1
  Gain9/1 -> Mux6/2
  Divide9/1 -> vbeta'/1
  Ibeta'/1 -> Mux6/4, Divide6/1, Divide6/2
  Ialpha'/1 -> Mux6/3, Divide5/1, Divide5/2
  Add8/1 -> Divide9/2, Divide8/2

== system final_1EHA_comfiltro_V9/EHA3/DSP/PLL ==
  Va : Inport
  Vb : Inport  Port=2
  Vc : Inport  Port=3
  Add10 : Sum
  Add3 : Sum  Inputs=+-
  Add4 : Sum  Inputs=+-
  Fcn1 : Fcn  Expr=sin(u(1))
  Fcn2 : Fcn  Expr=sin(u(1)+2*pi/3)
  Fcn3 : Fcn  Expr=sin(u(1)-pi/2)
  Fcn4 : Fcn  Expr=-cos(u(1)-pi/2)
  Integrator : Integrator
  PID Controller : simulink/Continuous/PID Controller  Controller=PI  TimeDomain=Continuous-time  SampleTime=-1  IntegratorMethod=Forward Euler  FilterMethod=Forward Euler  Form=Parallel  UseFilter=on  ControllerParametersSource=internal  P=25  I=22  D=0  N=100  InitialConditionSource=internal  InitialConditionForIntegrator=0  InitialConditionForFilter=0  ExternalReset=none  LimitOutput=off  UpperSaturationLimit=inf  LowerSaturationLimit=-inf  LinearizeAsGain=on  AntiWindupMode=none  Kb=1  TrackingMode=off  Kt=1  PParamMin=[]  PParamMax=[]  IParamMin=[]  IParamMax=[]  DParamMin=[]  DParamMax=[]  NParamMin=[]  NParamMax=[]  KbParamMin=[]  KbParamMax=[]  KtParamMin=[]  KtParamMax=[]  POutMin=[]  POutMax=[]  IOutMin=[]  IOutMax=[]  DOutMin=[]  DOutMax=[]  NOutMin=[]  NOutMax=[]  KbOutMin=[]  KbOutMax=[]  KtOutMin=[]  KtOutMax=[]  IntegratorOutMin=[]  IntegratorOutMax=[]  FilterOutMin=[]  FilterOutMax=[]  SumOutMin=[]  SumOutMax=[]  SumI1OutMin=[]  SumI1OutMax=[]  SumI2OutMin=[]  SumI2OutMax=[]  SumI3OutMin=[]  SumI3OutMax=[]  SumDOutMin=[]  SumDOutMax=[]  SaturationOutMin=[]  SaturationOutMax=[]  IntegratorContinuousStateAttributes=''  IntegratorStateMustResolveToSignalObject=off  IntegratorRTWStateStorageClass=Auto  FilterContinuousStateAttributes=''  FilterStateMustResolveToSignalObject=off  FilterRTWStateStorageClass=Auto  DifferentiatorICPrevScaledInput=0  DifferentiatorOutMin=[]  DifferentiatorOutMax=[]
  Product5 : Product
  Product6 : Product
  Ialpha' : Outport
  Ibeta' : Outport  Port=2
  wires:
  Va/1 -> Add3/1
  Add3/1 -> Product5/2  "Vab"
  Vc/1 -> Add4/1
  Fcn3/1 -> Ialpha'/1
  Fcn1/1 -> Product5/1
  Fcn2/1 -> Product6/2
  Integrator/1 -> Fcn2/1, Fcn4/1, Fcn1/1, Fcn3/1  "wt"
  Product6/1 -> Add10/2
  Vb/1 -> Add4/2, Add3/2
  Product5/1 -> Add10/1
  Add4/1 -> Product6/1  "Vcb"
  PID Controller/1 -> Integrator/1  "w"
  Add10/1 -> PID Controller/1  "P3phi"
  Fcn4/1 -> Ibeta'/1

== system final_1EHA_comfiltro_V9/EHA3/DSP/Subsystem ==
  Vabc' : Inport
  Iabc_L : Inport  Port=2
  Demux : Demux  Outputs=3
  Demux6 : Demux  Outputs=3
  Gain1 : Gain  Gain=sqrt(2/3)
  Gain2 : Gain  Gain=sqrt(2/3)
  Gain3 : Gain  Gain=[1/sqrt(2), 1/sqrt(2), 1/sqrt(2); 1, -1/2, -1/2; 0, sqrt(3)/2, -sqrt(3)/2]  Multiplication=Matrix(K*u)
  Gain4 : Gain  Gain=[1/sqrt(2), 1/sqrt(2), 1/sqrt(2); 1, -1/2, -1/2; 0, sqrt(3)/2, -sqrt(3)/2]  Multiplication=Matrix(K*u)
  Scope15 : Scope  NumInputPorts=2
  Terminator : Terminator
  Terminator1 : Terminator
  Valpha' : Outport
  Vbeta' : Outport  Port=2
  Ialpha : Outport  Port=3
  Ibeta : Outport  Port=4
  wires:
  Gain1/1 -> Gain3/1
  Gain2/1 -> Gain4/1
  Gain3/1 -> Demux/1, Scope15/1  "Valphabeta0"
  Demux/2 -> Valpha'/1  "Valpha"
  Demux6/2 -> Ialpha/1  "Ialpha"
  Demux/3 -> Vbeta'/1  "Vbeta"
  Demux6/3 -> Ibeta/1  "Ibeta"
  Iabc_L/1 -> Gain2/1
  Vabc'/1 -> Gain1/1
  Gain4/1 -> Demux6/1, Scope15/2  "Ialphabeta0"
  Demux6/1 -> Terminator/1  "I0"
  Demux/1 -> Terminator1/1  "V0"

== system final_1EHA_comfiltro_V9/EHA3/DSP/Subsystem1 ==
  Valpha' : Inport
  Vbeta' : Inport  Port=2
  Ialpha : Inport  Port=3
  Ibeta : Inport  Port=4
  Add : Sum
  Add10 : Sum
  Add3 : Sum  Inputs=+-
  Add4 : Sum  Inputs=+-
  LPF : dsparch4/Analog Filter Design  method=Butterworth  filttype=Lowpass  N=5  Wlo=2*pi*200  Whi=80  Rp=2  Rs=40
  Product{5..8} (4 alike) : Product
  Scope18 : Scope  NumInputPorts=5
  Posc : Outport
  q : Outport  Port=2
  wires:
  Product5/1 -> Add/1
  Product6/1 -> Add/2
  Add/1 -> Add4/2, LPF/1, Scope18/1  "P"
  Product7/1 -> Add3/1
  Product8/1 -> Add3/2
  Add3/1 -> q/1  "q"
  LPF/1 -> Add4/1, Scope18/2  "Pbarra"
  Vbeta'/1 -> Product7/1, Product6/1
  Ialpha/1 -> Product7/2, Product5/2
  Valpha'/1 -> Product8/1, Product5/1
  Ibeta/1 -> Product8/2, Product6/2
  Add10/1 -> Posc/1, Scope18/5  "Posc"
  Add4/1 -> Scope18/3, Add10/2  "-Ptil"
  [Ploss3] -> Scope18/4, Add10/1  "Ploss"

== system final_1EHA_comfiltro_V9/EHA3/DSP/Subsystem2 ==
  Valpha' : Inport
  Vbeta' : Inport  Port=2
  Posc : Inport  Port=3
  q : Inport  Port=4
  Add8 : Sum
  Add9 : Sum  Inputs=+-
  Divide{1..4} (4 alike) : Product  Inputs=***
  Fcn : Fcn  Expr=1/(u(1)^2+u(2)^2)
  Gain : Gain
  Gain5 : Gain  Gain=-1
  Mux : Mux  Inputs=2
  Scope20 : Scope  NumInputPorts=2
  Ialpha_p : Outport
  Ibeta_p : Outport  Port=2
  wires:
  Mux/1 -> Fcn/1
  Valpha'/1 -> Divide4/1, Mux/1, Divide1/1
  Vbeta'/1 -> Mux/2, Divide2/1, Divide3/1
  Posc/1 -> Gain5/1
  Fcn/1 -> Divide4/3, Divide3/3, Divide2/3, Divide1/3
  q/1 -> Gain/1
  Divide1/1 -> Add8/1
  Divide2/1 -> Add8/2
  Divide3/1 -> Add9/1
  Divide4/1 -> Add9/2
  Add9/1 -> Ibeta_p/1, Scope20/2  "Ibeta^*"
  Add8/1 -> Ialpha_p/1, Scope20/1  "Iaplha^*"
  Gain/1 -> Divide2/2, Divide4/2
  Gain5/1 -> Divide1/2, Divide3/2

== system final_1EHA_comfiltro_V9/EHA3/DSP/Subsystem3 ==
  Ialpha_p : Inport
  Ibeta_p : Inport  Port=2
  Fcn1 : Fcn  Expr=sqrt(2/3)*u(1)
  Fcn2 : Fcn  Expr=sqrt(2/3)*(-1/2*u(1)+sqrt(3)/2*u(2))
  Fcn3 : Fcn  Expr=sqrt(2/3)*(-1/2*u(1)-sqrt(3)/2*u(2))
  Mux2 : Mux  Inputs=2
  Mux3 : Mux  Inputs=2
  Mux5 : Mux  Inputs=2
  Scope14 : Scope  NumInputPorts=3
  Ia_C : Outport
  Ib_C : Outport  Port=2
  Ic_C : Outport  Port=3
  wires:
  Ibeta_p/1 -> Mux2/2, Mux3/2, Mux5/2
  Ialpha_p/1 -> Mux5/1, Mux2/1, Mux3/1
  Mux2/1 -> Fcn1/1
  Fcn1/1 -> Ia_C/1, Scope14/1  "Ia_C"
  Mux3/1 -> Fcn2/1
  Fcn2/1 -> Ib_C/1, Scope14/2  "Ib_C"
  Mux5/1 -> Fcn3/1
  Fcn3/1 -> Scope14/3, Ic_C/1  "Ic_C"

== system final_1EHA_comfiltro_V9/EHA3/DSP/TCT ==
  Va : Inport
  Vb : Inport  Port=2
  Vc : Inport  Port=3
  Demux7 : Demux  Outputs=3
  Gain1 : Gain  Gain=sqrt(2/3)
  Gain3 : Gain  Gain=[1/sqrt(2), 1/sqrt(2), 1/sqrt(2); 1, -1/2, -1/2; 0, sqrt(3)/2, -sqrt(3)/2]  Multiplication=Matrix(K*u)
  Mux2 : Mux  Inputs=3
  valpha : Outport
  vbeta : Outport  Port=2
  wires:
  Gain3/1 -> Demux7/1  "Valphabeta0"
  Gain1/1 -> Gain3/1
  Mux2/1 -> Gain1/1
  Va/1 -> Mux2/1
  Vb/1 -> Mux2/2
  Vc/1 -> Mux2/3
  Demux7/2 -> valpha/1
  Demux7/3 -> vbeta/1

== system final_1EHA_comfiltro_V9/EHA3/DSP/Transformada Inversa de Clarke ==
  valpha' : Inport
  vbeta' : Inport  Port=2
  Demux6 : Demux  Outputs=3
  Fcn10 : Fcn  Expr=sqrt(2/3)*(-1/2*u(1)+sqrt(3)/2*u(2))
  Fcn11 : Fcn  Expr=sqrt(2/3)*(-1/2*u(1)-sqrt(3)/2*u(2))
  Fcn9 : Fcn  Expr=sqrt(2/3)*(u(1) + 0*u(2))
  Mux{3,5,8..9} (4 alike) : Mux  Inputs=2
  Scope23 : Scope  NumInputPorts=3
  va' : Outport
  vb' : Outport  Port=2
  vc' : Outport  Port=3
  wires:
  Fcn10/1 -> vb'/1, Scope23/2  "vb'"
  Demux6/1 -> Mux9/1
  valpha'/1 -> Mux5/1, Mux8/1, Mux3/1
  vbeta'/1 -> Mux3/2, Mux5/2, Mux8/2
  Mux5/1 -> Fcn10/1
  Mux3/1 -> Fcn9/1
  Fcn11/1 -> vc'/1, Scope23/3  "vc'"
  Fcn9/1 -> va'/1, Mux9/2  "va'"
  Mux8/1 -> Fcn11/1
  [Vabc_S] -> Demux6/1
  Mux9/1 -> Scope23/1

== system final_1EHA_comfiltro_V9/EHA3/Inversor/Hysteresis controller ==
  I_ref : Inport
  I_meas : Inport  Port=2
  Demux2 : Demux  Outputs=3
  Demux3 : Demux  Outputs=3
  Logical Operator4 : Logic  Operator=NOT  AllPortsSameDT=off  OutDataTypeStr=boolean
  Logical Operator5 : Logic  Operator=NOT  AllPortsSameDT=off  OutDataTypeStr=boolean
  Logical Operator6 : Logic  Operator=NOT  AllPortsSameDT=off  OutDataTypeStr=boolean
  Memory : Memory
  Memory1 : Memory
  Mux3 : Mux  Inputs=6
  Relay : Relay  OnSwitchValue=0.05  OffSwitchValue=-0.05  OutDataTypeStr=Inherit: Inherit via back propagation
  Relay1 : Relay  OnSwitchValue=0.05  OffSwitchValue=-0.05  OutDataTypeStr=Inherit: Inherit via back propagation
  Relay2 : Relay  OnSwitchValue=0.05  OffSwitchValue=-0.05  OutDataTypeStr=Inherit: Inherit via back propagation
  Sum : Sum  Inputs=|+-
  Sum1 : Sum  Inputs=|+-
  Sum2 : Sum  Inputs=|+-
  g : Outport
  wires:
  I_ref/1 -> Memory/1
  I_meas/1 -> Memory1/1
  Relay1/1 -> Logical Operator5/1, Mux3/3
  Demux3/1 -> Sum/1
  Logical Operator4/1 -> Mux3/2
  Logical Operator5/1 -> Mux3/4
  Logical Operator6/1 -> Mux3/6
  Mux3/1 -> g/1
  Demux2/1 -> Sum/2
  Memory/1 -> Demux3/1
  Memory1/1 -> Demux2/1
  Relay/1 -> Mux3/1, Logical Operator4/1
  Demux3/2 -> Sum1/1
  Demux2/2 -> Sum1/2
  Demux3/3 -> Sum2/1
  Demux2/3 -> Sum2/2
  Relay2/1 -> Mux3/5, Logical Operator6/1
  Sum/1 -> Relay/1
  Sum1/1 -> Relay1/1
  Sum2/1 -> Relay2/1

== system final_1EHA_comfiltro_V9/EHA3/Inversor/PI controller ==
  Vdc : Inport
  LPF : dsparch4/Analog Filter Design  method=Butterworth  filttype=Lowpass  N=5  Wlo=2*pi*200  Whi=80  Rp=2  Rs=40
  PID Controller : simulink/Continuous/PID Controller  Controller=PI  TimeDomain=Continuous-time  SampleTime=-1  IntegratorMethod=Forward Euler  FilterMethod=Forward Euler  Form=Ideal  UseFilter=on  ControllerParametersSource=internal  P=5  I=7  D=0  N=100  InitialConditionSource=internal  InitialConditionForIntegrator=0  InitialConditionForFilter=0  ExternalReset=none  LimitOutput=off  UpperSaturationLimit=inf  LowerSaturationLimit=-inf  LinearizeAsGain=on  AntiWindupMode=none  Kb=1  TrackingMode=off  Kt=1  PParamMin=[]  PParamMax=[]  IParamMin=[]  IParamMax=[]  DParamMin=[]  DParamMax=[]  NParamMin=[]  NParamMax=[]  KbParamMin=[]  KbParamMax=[]  KtParamMin=[]  KtParamMax=[]  POutMin=[]  POutMax=[]  IOutMin=[]  IOutMax=[]  DOutMin=[]  DOutMax=[]  NOutMin=[]  NOutMax=[]  KbOutMin=[]  KbOutMax=[]  KtOutMin=[]  KtOutMax=[]  IntegratorOutMin=[]  IntegratorOutMax=[]  FilterOutMin=[]  FilterOutMax=[]  SumOutMin=[]  SumOutMax=[]  SumI1OutMin=[]  SumI1OutMax=[]  SumI2OutMin=[]  SumI2OutMax=[]  SumI3OutMin=[]  SumI3OutMax=[]  SumDOutMin=[]  SumDOutMax=[]  SaturationOutMin=[]  SaturationOutMax=[]  IntegratorContinuousStateAttributes=''  IntegratorStateMustResolveToSignalObject=off  IntegratorRTWStateStorageClass=Auto  FilterContinuousStateAttributes=''  FilterStateMustResolveToSignalObject=off  FilterRTWStateStorageClass=Auto  DifferentiatorICPrevScaledInput=0  DifferentiatorOutMin=[]  DifferentiatorOutMax=[]
  Scope : Scope  NumInputPorts=3
  Signal Builder1 : Subsystem  Tag=STV Subsys  LoadFcn=sigbuilder_block('load');  StartFcn=sigbuilder_block('start');  StopFcn=sigbuilder_block('stop');  ClipboardFcn=sigbuilder_block('clipboard');  mask(Sigbuilder block){}
      mask help: Simulink:masks:SigbuilderBlock_MD
      mask init:
      | if ~strcmp(get_param(bdroot(gcbh),'SimulationStatus'),'stopped') tuvar = sigbuilder_block('maskInit'); end
      settings: CopyFcn=sigbuilder_block('copy');  DeleteFcn=sigbuilder_block('delete');  ModelCloseFcn=sigbuilder_block('modelClose');  PreSaveFcn=sigbuilder_block('preSave');  PauseFcn=sigbuilder_block('pause');  ContinueFcn=sigbuilder_block('continue');  NameChangeFcn=sigbuilder_block('namechange');  OpenFcn=sigbuilder_block('open',[437.6 199.2 550.4 400 ]);  CloseFcn=sigbuilder_block('close');
      mask Display: plot(0, 0, 100, 100,[2, 2, 32, 32, 2], [68, 8, 8, 68, 68],[32, 2], [38, 38], [32, 19, 2],[53, 60, 44], [32, 17, 17, 2],[16, 16, 31, 31]);txt = getActiveGroup(gcbh);text(2, 100, txt,'verticalAlignment', 'top');
  Sum : Sum  Inputs=|-+
  Ploss : Outport
  wires:
  Vdc/1 -> Scope/1, Sum/1  "Vdc1"
  Sum/1 -> Scope/2, LPF/1  "Vdc1-step"
  Signal Builder1/1(Signal 1) -> Sum/2
  LPF/1 -> PID Controller/1
  PID Controller/1 -> Scope/3, Ploss/1

== system final_1EHA_comfiltro_V9/EHA1/Inversor/PI controller/Signal Builder1 ==
  Demux : Demux  Tag=STV Demux  Outputs=1
  FromWs : FromWorkspace  Tag=STV FromWs  VariableName=tuvar  SampleTime=0
      SigBuilderData=|
      | common.afterFinalStr = 'Extrapolate'
      | common.sampleTime = 0
      | dataSet.timeRange = [0 74]
      | dataSet.name = 'Group 1'
      | sbobj.Groups.Name = 'Group 1'
      | sbobj.Groups.Signals.Name = 'Signal 1'
      | sbobj.Groups.Signals.XData = [0 72.66 72.66 74]
      | sbobj.Groups.Signals.YData = [0 0 620 620]
      | sbobj.Groups.TimeRange = [0 74]
  Signal 1 : Outport  Tag=STV Outport
  wires:
  Demux/1 -> Signal 1/1
  FromWs/1 -> Demux/1

== system final_1EHA_comfiltro_V9/EHA2/Inversor/PI controller/Signal Builder1 ==
  Demux : Demux  Tag=STV Demux  Outputs=1
  FromWs : FromWorkspace  Tag=STV FromWs  VariableName=tuvar  SampleTime=0
      SigBuilderData=|
      | common.afterFinalStr = 'Extrapolate'
      | common.sampleTime = 0
      | dataSet.timeRange = [0 74]
      | dataSet.name = 'Group 1'
      | sbobj.Groups.Name = 'Group 1'
      | sbobj.Groups.Signals.Name = 'Signal 1'
      | sbobj.Groups.Signals.XData = [0 72.66 72.66 74]
      | sbobj.Groups.Signals.YData = [0 0 620 620]
      | sbobj.Groups.TimeRange = [0 74]
  Signal 1 : Outport  Tag=STV Outport
  wires:
  Demux/1 -> Signal 1/1
  FromWs/1 -> Demux/1

== system final_1EHA_comfiltro_V9/EHA3/Inversor/PI controller/Signal Builder1 ==
  Demux : Demux  Tag=STV Demux  Outputs=1
  FromWs : FromWorkspace  Tag=STV FromWs  VariableName=tuvar  SampleTime=0
      SigBuilderData=|
      | common.afterFinalStr = 'Extrapolate'
      | common.sampleTime = 0
      | dataSet.timeRange = [0 74]
      | dataSet.name = 'Group 1'
      | sbobj.Groups.Name = 'Group 1'
      | sbobj.Groups.Signals.Name = 'Signal 1'
      | sbobj.Groups.Signals.XData = [0 72.66 72.66 74]
      | sbobj.Groups.Signals.YData = [0 0 620 620]
      | sbobj.Groups.TimeRange = [0 74]
  Signal 1 : Outport  Tag=STV Outport
  wires:
  Demux/1 -> Signal 1/1
  FromWs/1 -> Demux/1
